simulink model "q4_ACE"  (R2025a)
settings: Solver=VariableStepAuto  StartTime=0.0  StopTime=900  RelTol=1e-3
settings Model: Creator=dtemu  LastModifiedBy=dtemu

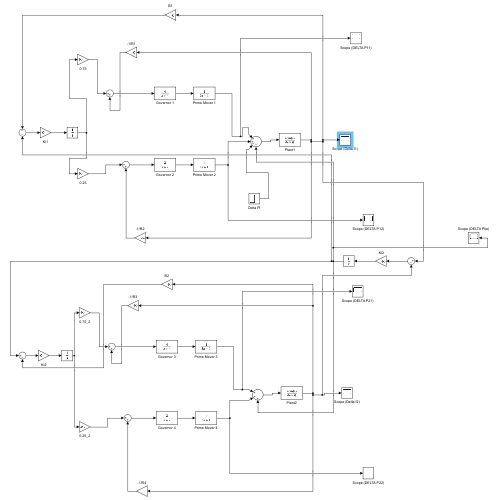
[thumbnail: Simulink's stored preview of the top-level diagram]
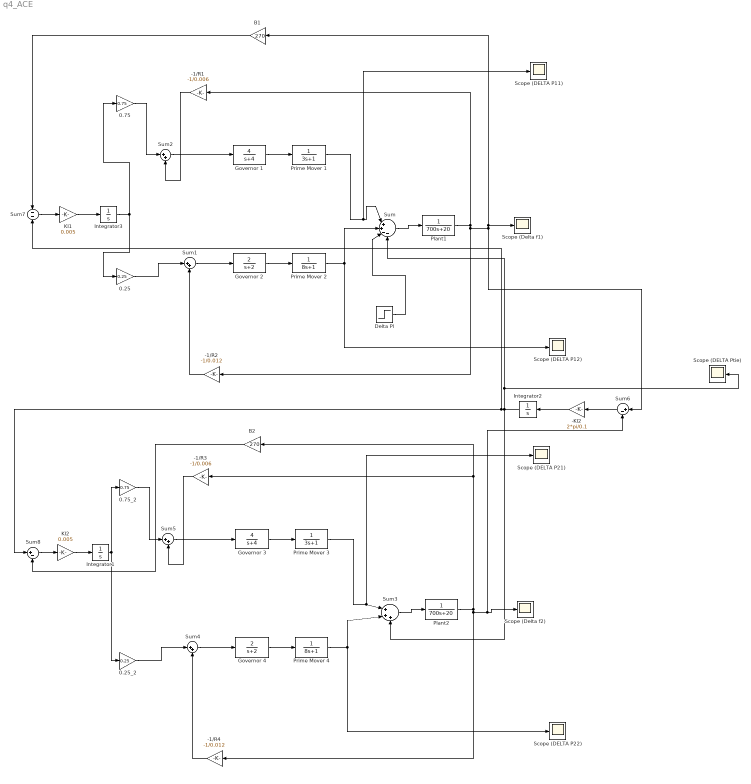
== system q4_ACE ==
  -1/R1 : Gain  Gain=-1/0.006
  -1/R2 : Gain  Gain=-1/0.012
  -1/R3 : Gain  Gain=-1/0.006
  -1/R4 : Gain  Gain=-1/0.012
  -KI2 : Gain  Gain=2*pi/0.1
  0.25 : Gain  Gain=0.25
  0.25_2 : Gain  Gain=0.25
  0.75 : Gain  Gain=0.75
  0.75_2 : Gain  Gain=0.75
  B1 : Gain  Gain=270
  B2 : Gain  Gain=270
  Delta Pl : Step  Time=0  After=100  SampleTime=0
  Governor 1 : TransferFcn  Numerator=[4]  Denominator=[1 4]
  Governor 2 : TransferFcn  Numerator=[2]  Denominator=[1 2]
  Governor 3 : TransferFcn  Numerator=[4]  Denominator=[1 4]
  Governor 4 : TransferFcn  Numerator=[2]  Denominator=[1 2]
  Integrator1 : Integrator
  Integrator2 : Integrator
  Integrator3 : Integrator
  KI1 : Gain  Gain=0.005
  KI2 : Gain  Gain=0.005
  Plant1 : TransferFcn  Denominator=[700 20]
  Plant2 : TransferFcn  Denominator=[700 20]
  Prime Mover 1 : TransferFcn  Denominator=[3 1]
  Prime Mover 2 : TransferFcn  Denominator=[8 1]
  Prime Mover 3 : TransferFcn  Denominator=[3 1]
  Prime Mover 4 : TransferFcn  Denominator=[8 1]
  Scope (DELTA P11) : Scope
      settings: ActiveDisplayYMinimum=-1  ActiveDisplayYMaximum=1  DataLoggingVariableName=ScopeData2
  Scope (DELTA P12) : Scope
      settings: ActiveDisplayYMinimum=-9.1343623216317518  ActiveDisplayYMaximum=39.336792897922535
  Scope (DELTA P21) : Scope
      settings: ActiveDisplayYMinimum=-6.2276951201791206  ActiveDisplayYMaximum=56.0492560816121  DataLoggingVariableName=ScopeData3
  Scope (DELTA P22) : Scope
      settings: ActiveDisplayYMinimum=-9.1343623216317518  ActiveDisplayYMaximum=39.336792897922535  DataLoggingVariableName=ScopeData4
  Scope (DELTA Ptie) : Scope
      settings: ActiveDisplayYMinimum=-81.717390808480133  ActiveDisplayYMaximum=9.0797100898311243  DataLoggingVariableName=ScopeData6
  Scope (Delta f1) : Scope
      settings: ActiveDisplayYMinimum=-0.4021831583821926  ActiveDisplayYMaximum=0.044687017598021392
  Scope (Delta f2) : Scope
      settings: ActiveDisplayYMinimum=-0.63110521231046024  ActiveDisplayYMaximum=0.0701228013678289  DataLoggingVariableName=ScopeData5
  Sum : Sum  Inputs=|++--
  Sum{1..2,4..5} (4 alike) : Sum  Inputs=|++
  Sum3 : Sum  Inputs=|+++
  Sum6 : Sum  Inputs=|+-
  Sum7 : Sum  Inputs=--
  Sum8 : Sum  Inputs=|+-
  wires:
  -KI2/1 -> Integrator2/1
  Governor 1/1 -> Prime Mover 1/1
  Sum/1 -> Plant1/1
  Sum2/1 -> Governor 1/1
  -1/R2/1 -> Sum1/2
  Governor 2/1 -> Prime Mover 2/1
  Sum1/1 -> Governor 2/1
  -1/R1/1 -> Sum2/2
  Plant1/1 -> B1/1, Scope (Delta f1)/1, Sum6/1, -1/R2/1, -1/R1/1
  Governor 3/1 -> Prime Mover 3/1
  Integrator2/1 -> Sum8/1, Sum7/2, Scope (DELTA Ptie)/1, Sum/4, Sum3/3
  Sum5/1 -> Governor 3/1
  Prime Mover 2/1 -> Scope (DELTA P12)/1, Sum/2
  0.25/1 -> Sum1/1
  Prime Mover 4/1 -> Scope (DELTA P22)/1, Sum3/2
  Sum6/1 -> -KI2/1
  Sum3/1 -> Plant2/1
  0.25_2/1 -> Sum4/1
  -1/R4/1 -> Sum4/2
  Sum4/1 -> Governor 4/1
  Delta Pl/1 -> Sum/3
  Prime Mover 3/1 -> Scope (DELTA P21)/1, Sum3/1
  Governor 4/1 -> Prime Mover 4/1
  0.75/1 -> Sum2/1
  -1/R3/1 -> Sum5/2
  0.75_2/1 -> Sum5/1
  Plant2/1 -> B2/1, -1/R3/1, Sum6/2, Scope (Delta f2)/1, -1/R4/1
  Prime Mover 1/1 -> Scope (DELTA P11)/1, Sum/1
  B1/1 -> Sum7/1
  Sum7/1 -> KI1/1
  KI1/1 -> Integrator3/1
  Integrator3/1 -> 0.25/1, 0.75/1
  B2/1 -> Sum8/2
  Sum8/1 -> KI2/1
  KI2/1 -> Integrator1/1
  Integrator1/1 -> 0.75_2/1, 0.25_2/1
